simulink model "lab2"  (R2015a)
settings: Solver=FixedStepDiscrete  StartTime=0.0  StopTime=20  RelTol=1e-3
values from neighbouring files (symbols this model uses):
  A = [1.37189711143 1 0 0 0 0 0.796247030428 0 1 0 0 0 ... (36 elements, 6x6)]    [matrizes.mat]
  B = [1 0 0 0 0 0]    [matrizes.mat]
  C = [0.176432501593 -0.307260665336 -0.097075632123 0.119078500307 -0.365349527089 0]    [matrizes.mat]
  D = 0    [matrizes.mat]
  K = [0.152892335406 -0.0494306399458 -0.17992491845 0.0741519455973 0.109452261993 -0.0633139239932]    [matrizes.mat]
  M = [-4.02099236255 -3.77131879733 -2.84355374965 -1.32107837653 -1.17257932747 0.607476554194]    [matrizes.mat]
  Nbar = -2.20135488168    [matrizes.mat]    (also in script_lab2.m = Nu+K*Nx)
undefined symbols (not defined in the file or in its folder): National_Instruments, PCI
libraries: sldrtlib x3
settings Model: SimulationMode=external  ExtModeTrigDuration=1000000  Creator=Alunos  LastModifiedBy=Alunos
settings HardwareCC: ProdIntDivRoundTo=Zero  ProdEndianess=LittleEndian  ProdHWDeviceType=Intel->x86/Pentium  TargetIntDivRoundTo=Zero  TargetEndianess=LittleEndian  TargetHWDeviceType=Intel->x86/Pentium
settings RTWCC: SystemTargetFile=rtwin.tlc  TemplateMakefile=rtwin.tmf  Description=Simulink Desktop Real-Time  RTWCompilerOptimization=on
settings CodeAppCC: MaxIdLength=95
settings RTWinTargetCC: TargetPreCompLibLocation=C:\Program Files\MATLAB\R2015a\toolbox\sldrt\lib\win32  ExtModeMexArgs=30

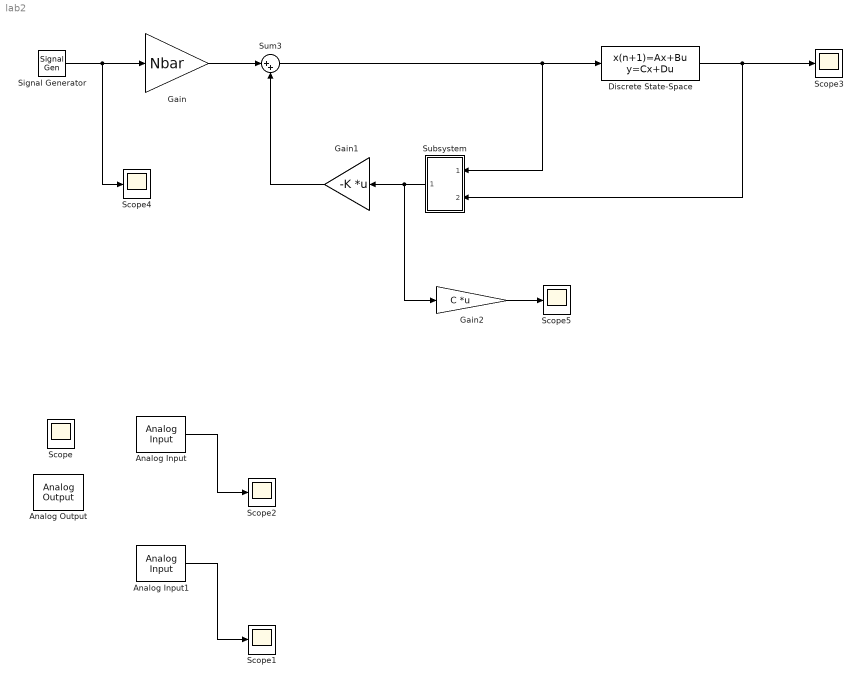
== system lab2 ==
  Analog Input : sldrtlib/Analog Input  SampleTime=0.02  MaxMissedTicks=10  ShowMissedTicks=off  YieldWhenWaiting=off  DrvName=National_Instruments/PCI-6221  DrvAddress=4294967295  DrvOptions=[0 0 0 0 0]  Channels=1  RangeMode=1  VoltRange=1  DataType=1
      settings: AttributesFormatString=National Instruments\nPCI-6221 [auto]
  Analog Input1 : sldrtlib/Analog Input  SampleTime=0.02  MaxMissedTicks=10  ShowMissedTicks=off  YieldWhenWaiting=off  DrvName=National_Instruments/PCI-6221  DrvAddress=4294967295  DrvOptions=[0 0 0 0 0]  Channels=2  RangeMode=1  VoltRange=1  DataType=1
      settings: AttributesFormatString=National Instruments\nPCI-6221 [auto]
  Analog Output : sldrtlib/Analog Output  SampleTime=0.02  MaxMissedTicks=10  ShowMissedTicks=off  YieldWhenWaiting=off  DrvName=National_Instruments/PCI-6221  DrvAddress=4294967295  DrvOptions=[0 0 0 0 0]  Channels=1  RangeMode=1  VoltRange=1  InitialValue=0  FinalValue=0
      settings: AttributesFormatString=National Instruments\nPCI-6221 [auto]
  Discrete State-Space : DiscreteStateSpace  A=A  B=B  C=C  D=D  SampleTime=0.02
  Gain : Gain  Gain=Nbar
  Gain1 : Gain  Gain=-K  Multiplication=Matrix(K*u) (u vector)
  Gain2 : Gain  Gain=C  Multiplication=Matrix(K*u) (u vector)
  Scope{,1..5} (6 alike) : Scope
      Scope settings: TickLabels=on  YMin=-10  YMax=10  SaveName=input  SampleInput=on
      Scope1 settings: SaveName=tensao_ext  SampleInput=on
      Scope2 settings: SaveName=tensao_pot  SampleInput=on
      Scope3 settings: SaveName=y_simulado
      Scope4 settings: SaveName=y_simulado1
      Scope5 settings: SaveName=y_simulado2
  Signal Generator : SignalGenerator  WaveForm=square  Frequency=0.2
  Subsystem : Subsystem
  Sum3 : Sum  Inputs=|++
  wires:
  Analog Input/1 -> Scope2/1
  Analog Input1/1 -> Scope1/1
  Sum3/1 -> Subsystem/1(In1), Discrete State-Space/1
  Gain/1 -> Sum3/1
  Gain1/1 -> Sum3/2
  Discrete State-Space/1 -> Scope3/1, Subsystem/2(In2)
  Subsystem/1(Out1) -> Gain2/1, Gain1/1
  Signal Generator/1 -> Scope4/1, Gain/1
  Gain2/1 -> Scope5/1

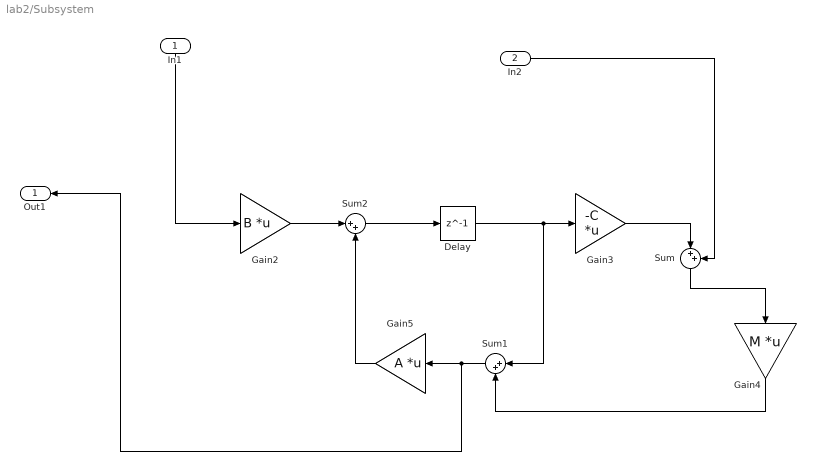
== system lab2/Subsystem ==
  In1 : Inport
  In2 : Inport  Port=2
  Delay : Delay  DelayLength=1  InitialCondition=0
  Gain2 : Gain  Gain=B  Multiplication=Matrix(K*u)
  Gain3 : Gain  Gain=-C  Multiplication=Matrix(K*u) (u vector)
  Gain4 : Gain  Gain=M  Multiplication=Matrix(K*u)
  Gain5 : Gain  Gain=A  Multiplication=Matrix(K*u) (u vector)
  Sum : Sum  Inputs=|++
  Sum1 : Sum  Inputs=|++
  Sum2 : Sum  Inputs=|++
  Out1 : Outport
  wires:
  Gain3/1 -> Sum/1
  In1/1 -> Gain2/1
  Gain4/1 -> Sum1/2
  Sum/1 -> Gain4/1
  Gain5/1 -> Sum2/2
  Sum1/1 -> Out1/1, Gain5/1
  In2/1 -> Sum/2
  Sum2/1 -> Delay/1
  Delay/1 -> Sum1/1, Gain3/1
  Gain2/1 -> Sum2/1
